simulink model "VFControl"  (R2017b)
settings: Solver=ode23tb  StartTime=0.0  StopTime=3  MaxStep=1e-4  RelTol=1e-3
undefined symbols (not defined in the file): DiscIntNeverNeededParam
libraries: simulink x5, powerlib x4
settings Model: Creator=80573  LastModifiedBy=80573
settings SolverCC: ZeroCrossAlgorithm=Adaptive
settings DebuggingCC: IgnoredZcDiagnostic=none

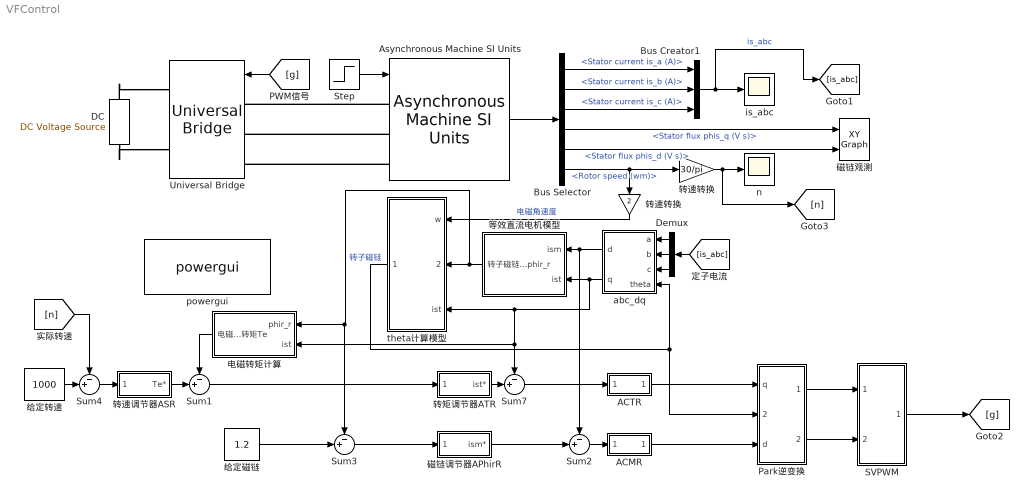
== system VFControl ==
  ACMR : Subsystem
  ACTR : Subsystem
  Asynchronous Machine SI Units : powerlib/Machines/Asynchronous Machine SI Units  RotorType=Squirrel-cage  PresetModel=No  MechanicalLoad=Torque Tm  ShowDetailedParameters=on  ReferenceFrame=Stationary  Units=SI  MeasurementBus=off  NominalParameters=[2200 380 50]  Stator=[0.435 0.002]  Rotor=[0.816 0.002]  Cage1=[0.4155 0.002066]  Cage2=[0.4168 0.0003495]  Lm=0.069  Mechanical=[0.19 0 2]  PolePairs=2  InitialConditions=[1 0 0 0 0 0 0 0]  SimulateSaturation=off  Saturation=[14.03593122, 27.81365428, 53.79336849, 72.68890987, 97.98006896, 148.6815601, 215.7428561, 302.9841135, 428.7778367 ; 230, 322, 414, 460, 506, 552, 598, 644, 690]  LoadFlowParameters=1492000  TsPowergui=0  TsBlock=-1  IterativeModel=Trapezoidal non iterative  IterativeDiscreteModel=Trapezoidal non iterative  Pmec=1.492e+006
  Bus Creator1 : BusCreator  Inputs=3
  Bus Selector : BusSelector  OutputSignals=Stator measurements.Stator current is_a (A),Stator measurements.Stator current is_b (A),Stator measurements.Stator current is_c (A),Stator measurements.Stator flux phis_q (V s),Stator measurements.Stator flux phis_d (V s),Mechanical.Rotor speed (wm)
  DC : powerlib/Electrical Sources/DC Voltage Source  Amplitude=510  Measurements=None
  Demux : Demux  Outputs=3
  Park逆变换 : Subsystem
  SVPWM : Subsystem
  Step : Step  Time=0.6  After=55  SampleTime=0
  Sum{1..4,7} (5 alike) : Sum  Inputs=-+|
  Universal Bridge : powerlib/Power Electronics/Universal Bridge  Arms=3  SnubberResistance=1e5  SnubberCapacitance=inf  Device=IGBT / Diodes  Ron=1e-3  Lon=0  ForwardVoltages="[  0  0  ]"  ForwardVoltage=0  GTOparameters=[ 10e-6 , 20e-6 ]  IGBTparameters=[ 1e-6 , 2e-6 ]  Measurements=None  Measurements_2=None  converterType=Rectifier
  abc_dq : Subsystem
  is_abc : Scope
  n : Scope
  powergui : powerlib/powergui  SimulationMode=Discrete  SampleTime=1e-5  frequency=50  Iterations=50  frequencyindice=50  Pbase=100e6  ErrMax=1e-4  UnitsV=kV  UnitsW=MW  buscounter=0  FunctionMessages=off  echomessages=off  EnableUseOfTLC=off  CurrentSourceSwitches=off  DisableSnubberDevices=off  DisableRonSwitches=off  DisableVfSwitches=off  DisplayEquations=off  SolverType=Tustin/Backward Euler (TBE)  Interpol=off  ExternalGateDelay=off  methode=off  Ts=100  x0status=zero  SPID=on  SwTol=0  HookPort=off  RestoreLinks=warning  ResistiveCurrentMeasurement=off  Frange=[0:2:500]  Ylog=off  Xlog=on  ShowGrid=off  save=off  variable=ZData  structure=0  ZoomFFT=on  StartTime=0.0  cycles=1  DisplayStyle=1  fundamental=60  FreqAxis=off  MaxFrequency=1000  frequencyindicesteady=1  RmsSteady=1  display=off
  theta计算模型 : Subsystem
  电磁转矩计算 : Subsystem
  磁链观测 : simulink/Sinks/XY Graph  xmin=-1  xmax=1  ymin=-1  ymax=1  st=-1
  磁链调节器APhirR : Subsystem
  等效直流电机模型 : Subsystem
  给定磁链 : Constant  Value=1.2
  给定转速 : Constant  Value=1000
  转矩调节器ATR : Subsystem
  转速调节器ASR : Subsystem
  转速转换 : Gain  Gain=30/pi
  "转速转换 " : Gain  Gain=2
  wires:
  Step/1 -> Asynchronous Machine SI Units/1
  "转速转换 "/1 -> theta计算模型/1(w)  "电磁角速度"
  转速转换/1 -> [n], n/1
  给定转速/1 -> Sum4/2
  [n] -> Sum4/1
  Sum1/1 -> 转矩调节器ATR/1(" ")
  theta计算模型/1(theta) -> Park逆变换/2(Theta), abc_dq/4(theta)
  Bus Selector/1 -> Bus Creator1/1  "<Stator current is_a (A)>"
  给定磁链/1 -> Sum3/2
  Bus Selector/4 -> 磁链观测/1  "<Stator flux phis_q (V s)>"
  转速调节器ASR/1(Te*) -> Sum1/2
  电磁转矩计算/1(电磁转矩Te) -> Sum1/1
  Demux/1 -> abc_dq/1(a)
  [is_abc] -> Demux/1
  等效直流电机模型/1(转子磁链phir_r) -> Sum3/1, 电磁转矩计算/1(phir_r), theta计算模型/2(phir_r)  "转子磁链"
  Bus Selector/5 -> 磁链观测/2  "<Stator flux phis_d (V s)>"
  Sum4/1 -> 转速调节器ASR/1("  ")
  [g] -> Universal Bridge/1
  Sum3/1 -> 磁链调节器APhirR/1(" ")
  Demux/2 -> abc_dq/2(b)
  Demux/3 -> abc_dq/3(c)
  SVPWM/1(PWM) -> [g]
  Bus Selector/3 -> Bus Creator1/3  "<Stator current is_c (A)>"
  abc_dq/2(q) -> Sum7/1, 电磁转矩计算/2(ist), theta计算模型/3(ist), 等效直流电机模型/2(ist)
  Bus Selector/6 -> 转速转换/1, "转速转换 "/1  "<Rotor speed (wm)>"
  Bus Selector/2 -> Bus Creator1/2  "<Stator current is_b (A)>"
  Asynchronous Machine SI Units/1 -> Bus Selector/1
  Bus Creator1/1 -> [is_abc], is_abc/1  "is_abc"
  abc_dq/1(d) -> Sum2/1, 等效直流电机模型/1(ism)
  转矩调节器ATR/1(ist*) -> Sum7/2
  磁链调节器APhirR/1(ism*) -> Sum2/2
  Sum2/1 -> ACMR/1("  ")
  Sum7/1 -> ACTR/1("  ")
  ACTR/1(" ") -> Park逆变换/1(q)
  ACMR/1(" ") -> Park逆变换/3(d)
  Park逆变换/1(alpha) -> SVPWM/1(Ualpha)
  Park逆变换/2(beta) -> SVPWM/2(Ubeta)
  connections:
  DC/LConn1 -- Universal Bridge/RConn2
  Asynchronous Machine SI Units/LConn3 -- Universal Bridge/LConn3
  DC/RConn1 -- Universal Bridge/RConn1
  Asynchronous Machine SI Units/LConn1 -- Universal Bridge/LConn1
  Asynchronous Machine SI Units/LConn2 -- Universal Bridge/LConn2

== system VFControl/ACMR ==
  "  " : Inport
  I积分放大倍数 : Gain  Gain=100
  PI输出限幅 : Saturate  UpperLimit=75  LowerLimit=-75
  P比例放大倍数 : Gain
  Scope : Scope  NumInputPorts=2
  Sum1 : Sum  Inputs=|++
  带限幅的连续积分 : Integrator  LimitOutput=on  UpperSaturationLimit=390  LowerSaturationLimit=-390
  " " : Outport
  wires:
  Sum1/1 -> PI输出限幅/1
  PI输出限幅/1 -> " "/1, Scope/1
  P比例放大倍数/1 -> Sum1/1
  I积分放大倍数/1 -> 带限幅的连续积分/1
  带限幅的连续积分/1 -> Scope/2, Sum1/2
  "  "/1 -> I积分放大倍数/1, P比例放大倍数/1

== system VFControl/ACTR ==
  "  " : Inport
  I积分放大倍数 : Gain  Gain=1200
  PI输出限幅 : Saturate  UpperLimit=380  LowerLimit=-380
  P比例放大倍数 : Gain  Gain=2
  Scope : Scope  NumInputPorts=2
  Sum1 : Sum  Inputs=|++
  带限幅的连续积分 : Integrator  LimitOutput=on  UpperSaturationLimit=400  LowerSaturationLimit=-400
  " " : Outport
  wires:
  Sum1/1 -> PI输出限幅/1
  PI输出限幅/1 -> " "/1, Scope/1
  P比例放大倍数/1 -> Sum1/1
  I积分放大倍数/1 -> 带限幅的连续积分/1
  带限幅的连续积分/1 -> Scope/2, Sum1/2
  "  "/1 -> I积分放大倍数/1, P比例放大倍数/1

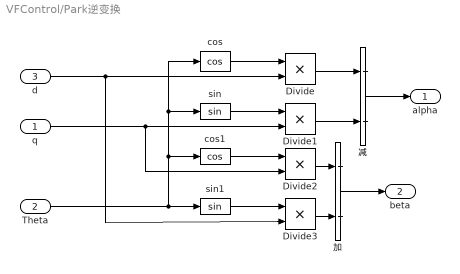
== system VFControl/Park逆变换 ==
  q : Inport
  Theta : Inport  Port=2
  d : Inport  Port=3
  Divide{,1..3} (4 alike) : Product  Inputs=**
  cos : Trigonometry  Operator=cos
  cos1 : Trigonometry  Operator=cos
  sin : Trigonometry
  sin1 : Trigonometry
  减 : Sum  Inputs=+-
  加 : Sum
  alpha : Outport
  beta : Outport  Port=2
  wires:
  sin/1 -> Divide1/1
  Divide2/1 -> 加/1
  cos1/1 -> Divide2/1
  cos/1 -> Divide/1
  Divide3/1 -> 加/2
  q/1 -> Divide2/2, Divide1/2
  Theta/1 -> cos/1, sin/1, cos1/1, sin1/1
  sin1/1 -> Divide3/1
  Divide1/1 -> 减/2
  Divide/1 -> 减/1
  d/1 -> Divide/2, Divide3/2
  加/1 -> beta/1
  减/1 -> alpha/1

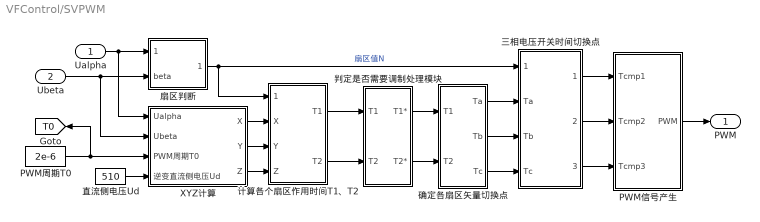
== system VFControl/SVPWM ==
  Ualpha : Inport
  Ubeta : Inport  Port=2
  PWM信号产生 : Subsystem
  PWM周期T0 : Constant  Value=2e-6
  XYZ计算 : Subsystem
  三相电压开关时间切换点 : Subsystem
  判定是否需要调制处理模块 : Subsystem
  扇区判断 : Subsystem
  直流侧电压Ud : Constant  Value=510
  确定各扇区矢量切换点 : Subsystem
  计算各个扇区作用时间T1、T2 : Subsystem
  PWM : Outport
  tag scope: T0=global
  wires:
  Ubeta/1 -> XYZ计算/2(Ubeta), 扇区判断/2(beta)
  Ualpha/1 -> XYZ计算/1(Ualpha), 扇区判断/1(alpha)
  PWM周期T0/1 -> XYZ计算/3(PWM周期T0), [T0]
  直流侧电压Ud/1 -> XYZ计算/4(逆变直流侧电压Ud)
  扇区判断/1(扇区值N) -> 计算各个扇区作用时间T1、T2/1(扇区值N), 三相电压开关时间切换点/1(扇区值N)  "扇区值N"
  XYZ计算/1(X) -> 计算各个扇区作用时间T1、T2/2(X)
  XYZ计算/2(Y) -> 计算各个扇区作用时间T1、T2/3(Y)
  XYZ计算/3(Z) -> 计算各个扇区作用时间T1、T2/4(Z)
  确定各扇区矢量切换点/2(Tb) -> 三相电压开关时间切换点/3(Tb)
  确定各扇区矢量切换点/3(Tc) -> 三相电压开关时间切换点/4(Tc)
  计算各个扇区作用时间T1、T2/2(T2) -> 判定是否需要调制处理模块/2(T2)
  计算各个扇区作用时间T1、T2/1(T1) -> 判定是否需要调制处理模块/1(T1)
  判定是否需要调制处理模块/2(T2*) -> 确定各扇区矢量切换点/2(T2)
  确定各扇区矢量切换点/1(Ta) -> 三相电压开关时间切换点/2(Ta)
  判定是否需要调制处理模块/1(T1*) -> 确定各扇区矢量切换点/1(T1)
  三相电压开关时间切换点/1(Tcmp1) -> PWM信号产生/1(Tcmp1)
  三相电压开关时间切换点/2(Tcmp2) -> PWM信号产生/2(Tcmp2)
  三相电压开关时间切换点/3(Tcmp3) -> PWM信号产生/3(Tcmp3)
  PWM信号产生/1(PWM) -> PWM/1

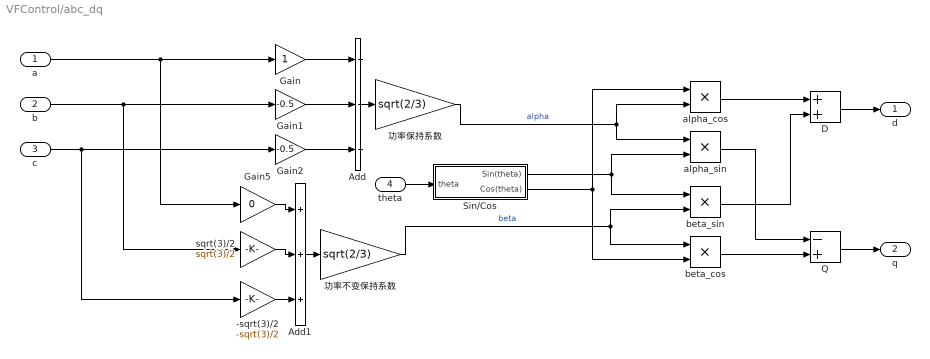
== system VFControl/abc_dq ==
  a : Inport
  b : Inport  Port=2
  c : Inport  Port=3
  theta : Inport  Port=4
  -sqrt(3)/2 : Gain  Gain=-sqrt(3)/2
  Add : Sum  Inputs=3
  Add1 : Sum  Inputs=3
  D : Sum
  Gain : Gain
  Gain1 : Gain  Gain=-0.5
  Gain2 : Gain  Gain=-0.5
  Gain5 : Gain  Gain=0
  Q : Sum  Inputs=-+
  Sin/Cos : Subsystem
  alpha_cos : Product
  alpha_sin : Product
  beta_cos : Product
  beta_sin : Product
  sqrt(3)/2 : Gain  Gain=sqrt(3)/2
  功率不变保持系数 : Gain  Gain=sqrt(2/3)
  功率保持系数 : Gain  Gain=sqrt(2/3)
  d : Outport
  q : Outport  Port=2
  wires:
  功率不变保持系数/1 -> beta_cos/1, beta_sin/2  "beta"
  D/1 -> d/1
  Sin/Cos/2(Cos(theta)) -> beta_cos/2, alpha_cos/1
  alpha_sin/1 -> Q/1
  Q/1 -> q/1
  beta_sin/1 -> D/2
  beta_cos/1 -> Q/2
  Sin/Cos/1(Sin(theta)) -> beta_sin/1, alpha_sin/2
  功率保持系数/1 -> alpha_cos/2, alpha_sin/1  "alpha"
  Add1/1 -> 功率不变保持系数/1
  c/1 -> Gain2/1, -sqrt(3)/2/1
  a/1 -> Gain5/1, Gain/1
  Gain2/1 -> Add/3
  sqrt(3)/2/1 -> Add1/2
  theta/1 -> Sin/Cos/1(theta)
  b/1 -> sqrt(3)/2/1, Gain1/1
  -sqrt(3)/2/1 -> Add1/3
  Gain1/1 -> Add/2
  Gain5/1 -> Add1/1
  alpha_cos/1 -> D/1
  Add/1 -> 功率保持系数/1
  Gain/1 -> Add/1

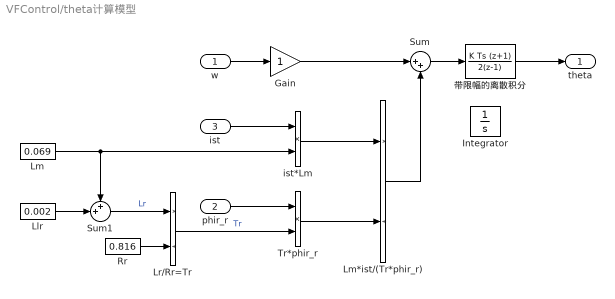
== system VFControl/theta计算模型 ==
  w : Inport
  phir_r : Inport  Port=2
  ist : Inport  Port=3
  Gain : Gain
  Integrator : Integrator
  Llr : Constant  Value=0.002
  Lm : Constant  Value=0.069
  Lm*ist/(Tr*phir_r) : Product  Inputs=*/
  Lr/Rr=Tr : Product  Inputs=*/
  Rr : Constant  Value=0.816
  Sum : Sum  Inputs=|++
  Sum1 : Sum  Inputs=++|
  Tr*phir_r : Product
  ist*Lm : Product
  带限幅的离散积分 : DiscreteIntegrator  IntegratorMethod=Integration: Trapezoidal  SampleTime=2e-5  LimitOutput=on  UpperSaturationLimit=3000  LowerSaturationLimit=-3000  ICPrevOutput=DiscIntNeverNeededParam  ICPrevScaledInput=DiscIntNeverNeededParam
  theta : Outport
  wires:
  ist*Lm/1 -> Lm*ist/(Tr*phir_r)/1
  Lm*ist/(Tr*phir_r)/1 -> Sum/2
  Sum/1 -> 带限幅的离散积分/1
  w/1 -> Gain/1
  带限幅的离散积分/1 -> theta/1
  Lr/Rr=Tr/1 -> Tr*phir_r/2  "Tr"
  Lm/1 -> Sum1/1, ist*Lm/2
  Tr*phir_r/1 -> Lm*ist/(Tr*phir_r)/2
  ist/1 -> ist*Lm/1
  phir_r/1 -> Tr*phir_r/1
  Rr/1 -> Lr/Rr=Tr/2
  Gain/1 -> Sum/1
  Sum1/1 -> Lr/Rr=Tr/1  "Lr"
  Llr/1 -> Sum1/2

== system VFControl/电磁转矩计算 ==
  phir_r : Inport
  ist : Inport  Port=2
  Llr : Constant  Value=0.002
  Lm : Constant  Value=0.069
  Sum1 : Sum  Inputs=++|
  ist*Lm*phir_r*np : Product  Inputs=4
  np : Constant  Value=2
  除法 : Product  Inputs=*/
  电磁转矩Te : Outport
  wires:
  np/1 -> ist*Lm*phir_r*np/4
  phir_r/1 -> ist*Lm*phir_r*np/3
  除法/1 -> 电磁转矩Te/1
  ist*Lm*phir_r*np/1 -> 除法/1
  Sum1/1 -> 除法/2  "Lr"
  Llr/1 -> Sum1/2
  ist/1 -> ist*Lm*phir_r*np/2
  Lm/1 -> Sum1/1, ist*Lm*phir_r*np/1

== system VFControl/磁链调节器APhirR ==
  " " : Inport
  I积分放大倍数 : Gain  Gain=100
  PI输出限幅 : Saturate  UpperLimit=13  LowerLimit=-13
  P比例放大倍数 : Gain  Gain=1.8
  Scope : Scope  NumInputPorts=2
  Sum1 : Sum  Inputs=|++
  带限幅的离散积分 : DiscreteIntegrator  SampleTime=2e-5  ICPrevOutput=DiscIntNeverNeededParam  ICPrevScaledInput=DiscIntNeverNeededParam
  带限幅的连续积分 : Integrator  LimitOutput=on  UpperSaturationLimit=15  LowerSaturationLimit=-15
  ism* : Outport
  wires:
  Sum1/1 -> PI输出限幅/1
  I积分放大倍数/1 -> 带限幅的连续积分/1
  P比例放大倍数/1 -> Sum1/1
  " "/1 -> I积分放大倍数/1, P比例放大倍数/1
  PI输出限幅/1 -> ism*/1, Scope/1
  带限幅的连续积分/1 -> Scope/2, Sum1/2

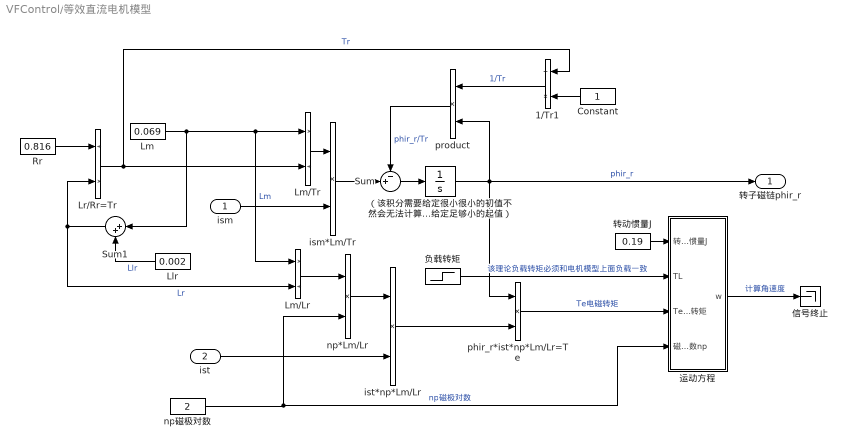
== system VFControl/等效直流电机模型 ==
  ism : Inport
  ist : Inport  Port=2
  1/Tr1 : Product  Inputs=/*
  Constant : Constant
  Llr : Constant  Value=0.002
  Lm : Constant  Value=0.069
  Lm/Lr : Product  Inputs=*/
  Lm/Tr : Product  Inputs=*/
  Lr/Rr=Tr : Product  Inputs=/*
  Rr : Constant  Value=0.816
  Sum : Sum  Inputs=-+|
  Sum1 : Sum  Inputs=|++
  ism*Lm/Tr : Product
  ist*np*Lm/Lr : Product
  np*Lm/Lr : Product
  np磁极对数 : Constant  Value=2
  phir_r*ist*np*Lm/Lr=Te : Product
  product : Product
  信号终止 : Terminator
  负载转矩 : Step  Time=0.6  After=55  SampleTime=0
  转动惯量J : Constant  Value=0.19
  运动方程 : Subsystem
  （该积分需要给定很小很小的初值不然会无法计算 原因是数学推导中积分起值为0所以一直都为0 所以要能够计算必须给定足够小的起值） : Integrator  InitialCondition=1e-5
  转子磁链phir_r : Outport
  wires:
  ism/1 -> ism*Lm/Tr/2
  Sum/1 -> （该积分需要给定很小很小的初值不然会无法计算 原因是数学推导中积分起值为0所以一直都为0 所以要能够计算必须给定足够小的起值）/1
  转动惯量J/1 -> 运动方程/1(转动惯量J)
  运动方程/1(w) -> 信号终止/1  "计算角速度"
  phir_r*ist*np*Lm/Lr=Te/1 -> 运动方程/3(Te电磁转矩)  "Te电磁转矩"
  负载转矩/1 -> 运动方程/2(TL)  "该理论负载转矩必须和电机模型上面负载一致"
  np*Lm/Lr/1 -> ist*np*Lm/Lr/1
  Lm/1 -> Sum1/1, Lm/Lr/1, Lm/Tr/1  "Lm"
  Lm/Tr/1 -> ism*Lm/Tr/1
  ist*np*Lm/Lr/1 -> phir_r*ist*np*Lm/Lr=Te/2
  ism*Lm/Tr/1 -> Sum/2
  product/1 -> Sum/1  "phir_r/Tr"
  ist/1 -> ist*np*Lm/Lr/2
  np磁极对数/1 -> np*Lm/Lr/2, 运动方程/4(磁极对数np)  "np磁极对数"
  Lm/Lr/1 -> np*Lm/Lr/1
  （该积分需要给定很小很小的初值不然会无法计算 原因是数学推导中积分起值为0所以一直都为0 所以要能够计算必须给定足够小的起值）/1 -> 转子磁链phir_r/1, product/2, phir_r*ist*np*Lm/Lr=Te/1  "phir_r"
  1/Tr1/1 -> product/1  "1/Tr"
  Lr/Rr=Tr/1 -> Lm/Tr/2, 1/Tr1/1  "Tr"
  Rr/1 -> Lr/Rr=Tr/1
  Constant/1 -> 1/Tr1/2
  Sum1/1 -> Lm/Lr/2, Lr/Rr=Tr/2  "Lr"
  Llr/1 -> Sum1/2  "Llr"

== system VFControl/转矩调节器ATR ==
  " " : Inport
  I积分放大倍数 : Gain  Gain=12
  PI输出限幅 : Saturate  UpperLimit=60  LowerLimit=-60
  P比例放大倍数 : Gain  Gain=4.5
  Scope : Scope  NumInputPorts=2
  Sum3 : Sum  Inputs=|++
  带限幅的离散积分 : DiscreteIntegrator  SampleTime=2e-5  ICPrevOutput=DiscIntNeverNeededParam  ICPrevScaledInput=DiscIntNeverNeededParam
  带限幅的连续积分 : Integrator  LimitOutput=on  UpperSaturationLimit=65  LowerSaturationLimit=-65
  ist* : Outport
  wires:
  Sum3/1 -> PI输出限幅/1
  P比例放大倍数/1 -> Sum3/1
  " "/1 -> I积分放大倍数/1, P比例放大倍数/1
  I积分放大倍数/1 -> 带限幅的连续积分/1
  PI输出限幅/1 -> ist*/1, Scope/1
  带限幅的连续积分/1 -> Scope/2, Sum3/2

== system VFControl/转速调节器ASR ==
  "  " : Inport
  I积分放大倍数 : Gain  Gain=0.8
  PI输出限幅 : Saturate  UpperLimit=75  LowerLimit=-75
  P比例放大倍数 : Gain  Gain=5
  Scope : Scope  NumInputPorts=2
  Sum1 : Sum  Inputs=|++
  带限幅的连续积分 : Integrator  LimitOutput=on  UpperSaturationLimit=80  LowerSaturationLimit=-80
  Te* : Outport
  wires:
  Sum1/1 -> PI输出限幅/1
  PI输出限幅/1 -> Te*/1, Scope/1
  P比例放大倍数/1 -> Sum1/1
  I积分放大倍数/1 -> 带限幅的连续积分/1
  带限幅的连续积分/1 -> Scope/2, Sum1/2
  "  "/1 -> I积分放大倍数/1, P比例放大倍数/1

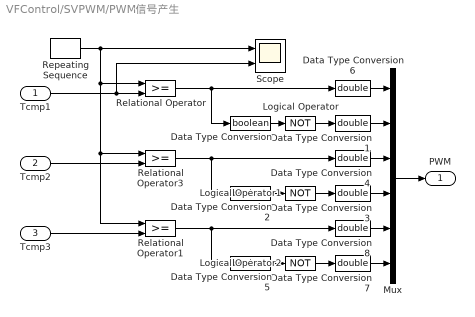
== system VFControl/SVPWM/PWM信号产生 ==
  Tcmp1 : Inport
  Tcmp2 : Inport  Port=2
  Tcmp3 : Inport  Port=3
  Data Type Conversion : DataTypeConversion  OutDataTypeStr=boolean
  Data Type Conversion{1,3..4,6..8} (6 alike) : DataTypeConversion  OutDataTypeStr=double
  Data Type Conversion2 : DataTypeConversion  OutDataTypeStr=boolean
  Data Type Conversion5 : DataTypeConversion  OutDataTypeStr=boolean
  Logical Operator : Logic  Operator=NOT  AllPortsSameDT=off  OutDataTypeStr=boolean
  Logical Operator1 : Logic  Operator=NOT  AllPortsSameDT=off  OutDataTypeStr=boolean
  Logical Operator2 : Logic  Operator=NOT  AllPortsSameDT=off  OutDataTypeStr=boolean
  Mux : Mux  Inputs=6
  Relational Operator : RelationalOperator  OutDataTypeStr=boolean  RndMeth=Nearest
  Relational Operator1 : RelationalOperator  OutDataTypeStr=boolean  RndMeth=Nearest
  Relational Operator3 : RelationalOperator  OutDataTypeStr=boolean  RndMeth=Nearest
  Repeating Sequence : simulink/Sources/Repeating Sequence  rep_seq_t=[0 1e-4 2e-4]  rep_seq_y=[0 1.3e-6 0]
  Scope : Scope  NumInputPorts=2
  PWM : Outport
  wires:
  Data Type Conversion/1 -> Logical Operator/1
  Logical Operator/1 -> Data Type Conversion1/1
  Relational Operator/1 -> Data Type Conversion6/1, Data Type Conversion/1
  Logical Operator1/1 -> Data Type Conversion3/1
  Relational Operator3/1 -> Data Type Conversion4/1, Data Type Conversion2/1
  Data Type Conversion2/1 -> Logical Operator1/1
  Relational Operator1/1 -> Data Type Conversion8/1, Data Type Conversion5/1
  Data Type Conversion5/1 -> Logical Operator2/1
  Logical Operator2/1 -> Data Type Conversion7/1
  Repeating Sequence/1 -> Relational Operator1/1, Relational Operator3/1, Relational Operator/1, Scope/1
  Tcmp1/1 -> Scope/2, Relational Operator/2
  Tcmp2/1 -> Relational Operator3/2
  Tcmp3/1 -> Relational Operator1/2
  Data Type Conversion6/1 -> Mux/1
  Data Type Conversion1/1 -> Mux/2
  Data Type Conversion4/1 -> Mux/3
  Data Type Conversion3/1 -> Mux/4
  Data Type Conversion8/1 -> Mux/5
  Data Type Conversion7/1 -> Mux/6
  Mux/1 -> PWM/1

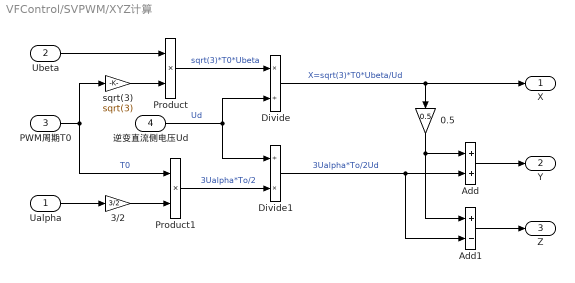
== system VFControl/SVPWM/XYZ计算 ==
  Ualpha : Inport
  Ubeta : Inport  Port=2
  PWM周期T0 : Inport  Port=3
  逆变直流侧电压Ud : Inport  Port=4
  0.5 : Gain  Gain=0.5
  3/2 : Gain  Gain=3/2
  Add : Sum
  Add1 : Sum  Inputs=+-
  Divide : Product  Inputs=*/
  Divide1 : Product  Inputs=/*
  Product : Product
  Product1 : Product
  "sqrt(3) " : Gain  Gain=sqrt(3)
  X : Outport
  Y : Outport  Port=2
  Z : Outport  Port=3
  wires:
  Divide/1 -> 0.5/1, X/1  "X=sqrt(3)*T0*Ubeta/Ud"
  Product/1 -> Divide/1  "sqrt(3)*T0*Ubeta"
  逆变直流侧电压Ud/1 -> Divide1/1, Divide/2  "Ud"
  Ualpha/1 -> 3/2/1
  Divide1/1 -> Add1/2, Add/2  "3Ualpha*To/2Ud"
  Add/1 -> Y/1
  Ubeta/1 -> Product/1
  3/2/1 -> Product1/2
  Product1/1 -> Divide1/2  "3Ualpha*To/2"
  "sqrt(3) "/1 -> Product/2
  PWM周期T0/1 -> "sqrt(3) "/1, Product1/1  "T0"
  Add1/1 -> Z/1
  0.5/1 -> Add/1, Add1/1

== system VFControl/SVPWM/三相电压开关时间切换点 ==
  扇区值N : Inport
  Ta : Inport  Port=2
  Tb : Inport  Port=3
  Tc : Inport  Port=4
  Multiport Switch : MultiPortSwitch  Inputs=6  OutDataTypeStr=double
  Multiport Switch1 : MultiPortSwitch  Inputs=6  OutDataTypeStr=double
  Multiport Switch2 : MultiPortSwitch  Inputs=6  OutDataTypeStr=double
  Tcmp1 : Outport
  Tcmp2 : Outport  Port=2
  Tcmp3 : Outport  Port=3
  wires:
  扇区值N/1 -> Multiport Switch2/1, Multiport Switch1/1, Multiport Switch/1  "扇区选择"
  Multiport Switch/1 -> Tcmp1/1
  Multiport Switch1/1 -> Tcmp2/1
  Multiport Switch2/1 -> Tcmp3/1
  Ta/1 -> Multiport Switch/4, Multiport Switch2/7, Multiport Switch2/5, Multiport Switch1/6, Multiport Switch1/2, Multiport Switch/3
  Tb/1 -> Multiport Switch2/6, Multiport Switch2/3, Multiport Switch1/5, Multiport Switch1/4, Multiport Switch/7, Multiport Switch/2
  Tc/1 -> Multiport Switch1/7, Multiport Switch2/2, Multiport Switch2/4, Multiport Switch1/3, Multiport Switch/6, Multiport Switch/5

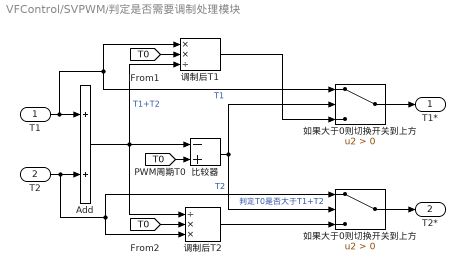
== system VFControl/SVPWM/判定是否需要调制处理模块 ==
  T1 : Inport
  T2 : Inport  Port=2
  Add : Sum
  如果大于0则切换开关到上方 : Switch  Criteria=u2 > Threshold
  "如果大于0则切换开关到上方 " : Switch  Criteria=u2 > Threshold
  比较器 : Sum  Inputs=-+
  调制后T1 : Product  Inputs=**/
  调制后T2 : Product  Inputs=/**
  T1* : Outport
  T2* : Outport  Port=2
  wires:
  如果大于0则切换开关到上方/1 -> T1*/1
  "如果大于0则切换开关到上方 "/1 -> T2*/1
  T2/1 -> "如果大于0则切换开关到上方 "/1, 调制后T2/3, Add/2  "T2"
  T1/1 -> 如果大于0则切换开关到上方/1, 调制后T1/1, Add/1  "T1"
  [T0] -> 比较器/2
  Add/1 -> 调制后T2/1, 比较器/1, 调制后T1/3  "T1+T2"
  比较器/1 -> "如果大于0则切换开关到上方 "/2, 如果大于0则切换开关到上方/2  "判定T0是否大于T1+T2"
  调制后T2/1 -> "如果大于0则切换开关到上方 "/3
  调制后T1/1 -> 如果大于0则切换开关到上方/3
  [T0] -> 调制后T1/2
  [T0] -> 调制后T2/2

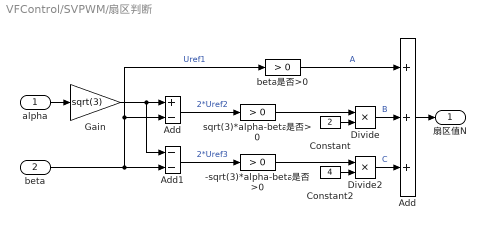
== system VFControl/SVPWM/扇区判断 ==
  alpha : Inport
  beta : Inport  Port=2
  -sqrt(3)*alpha-beta是否>0 : simulink/Logic and Bit Operations/Compare To Zero  relop=>  OutDataTypeStr=boolean
  Add : Sum  Inputs=+-
  "Add " : Sum  Inputs=+++
  Add1 : Sum  Inputs=--
  Constant : Constant  Value=2
  Constant2 : Constant  Value=4
  Divide : Product  Inputs=**
  Divide2 : Product  Inputs=**
  Gain : Gain  Gain=sqrt(3)
  beta是否>0 : simulink/Logic and Bit Operations/Compare To Zero  relop=>  OutDataTypeStr=boolean
  sqrt(3)*alpha-beta是否>0 : simulink/Logic and Bit Operations/Compare To Zero  relop=>  OutDataTypeStr=boolean
  扇区值N : Outport
  wires:
  beta/1 -> Add1/2, Add/2, beta是否>0/1  "Uref1"
  alpha/1 -> Gain/1
  Gain/1 -> Add/1, Add1/1
  Add/1 -> sqrt(3)*alpha-beta是否>0/1  "2*Uref2"
  Add1/1 -> -sqrt(3)*alpha-beta是否>0/1  "2*Uref3"
  -sqrt(3)*alpha-beta是否>0/1 -> Divide2/1
  sqrt(3)*alpha-beta是否>0/1 -> Divide/1
  Constant/1 -> Divide/2
  Constant2/1 -> Divide2/2
  beta是否>0/1 -> "Add "/1  "A"
  Divide/1 -> "Add "/2  "B"
  Divide2/1 -> "Add "/3  "C"
  "Add "/1 -> 扇区值N/1

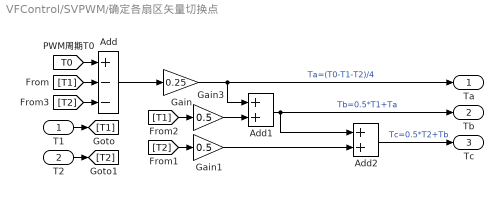
== system VFControl/SVPWM/确定各扇区矢量切换点 ==
  T1 : Inport
  T2 : Inport  Port=2
  Add : Sum  Inputs=+--
  Add1 : Sum
  Add2 : Sum
  Gain : Gain  Gain=0.25
  Gain1 : Gain  Gain=0.5
  Gain3 : Gain  Gain=0.5
  Ta : Outport
  Tb : Outport  Port=2
  Tc : Outport  Port=3
  wires:
  Gain/1 -> Ta/1, Add1/1  "Ta=(T0-T1-T2)/4"
  [T0] -> Add/1
  Add/1 -> Gain/1
  Add1/1 -> Tb/1, Add2/1  "Tb=0.5*T1+Ta"
  Add2/1 -> Tc/1  "Tc=0.5*T2+Tb"
  Gain3/1 -> Add1/2
  Gain1/1 -> Add2/2
  T1/1 -> [T1]
  [T1] -> Add/2
  T2/1 -> [T2]
  [T1] -> Gain3/1
  [T2] -> Gain1/1
  [T2] -> Add/3

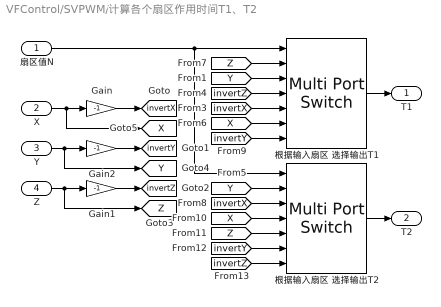
== system VFControl/SVPWM/计算各个扇区作用时间T1、T2 ==
  扇区值N : Inport
  X : Inport  Port=2
  Y : Inport  Port=3
  Z : Inport  Port=4
  Gain : Gain  Gain=-1
  Gain1 : Gain  Gain=-1
  Gain2 : Gain  Gain=-1
  根据输入扇区 选择输出T1 : MultiPortSwitch  Inputs=6
  根据输入扇区 选择输出T2 : MultiPortSwitch  Inputs=6
  T1 : Outport
  T2 : Outport  Port=2
  tag scope: X=global, Y=global, Z=global, invertX=global, invertY=global, invertZ=global
  wires:
  Z/1 -> [Z], Gain1/1
  X/1 -> [X], Gain/1
  扇区值N/1 -> 根据输入扇区 选择输出T2/1, 根据输入扇区 选择输出T1/1
  根据输入扇区 选择输出T2/1 -> T2/1
  根据输入扇区 选择输出T1/1 -> T1/1
  Y/1 -> [Y], Gain2/1
  Gain/1 -> [invertX]
  Gain2/1 -> [invertY]
  Gain1/1 -> [invertZ]
  [Z] -> 根据输入扇区 选择输出T1/2
  [Y] -> 根据输入扇区 选择输出T2/2
  [Y] -> 根据输入扇区 选择输出T1/3
  [invertX] -> 根据输入扇区 选择输出T2/3
  [invertZ] -> 根据输入扇区 选择输出T1/4
  [invertX] -> 根据输入扇区 选择输出T1/5
  [X] -> 根据输入扇区 选择输出T1/6
  [invertY] -> 根据输入扇区 选择输出T1/7
  [X] -> 根据输入扇区 选择输出T2/4
  [Z] -> 根据输入扇区 选择输出T2/5
  [invertY] -> 根据输入扇区 选择输出T2/6
  [invertZ] -> 根据输入扇区 选择输出T2/7

== system VFControl/abc_dq/Sin//Cos ==
  theta : Inport
  cos : Trigonometry  Operator=cos
  sin : Trigonometry
  Sin(theta) : Outport
  Cos(theta) : Outport  Port=2
  wires:
  sin/1 -> Sin(theta)/1
  theta/1 -> sin/1, cos/1
  cos/1 -> Cos(theta)/1

== system VFControl/等效直流电机模型/运动方程 ==
  转动惯量J : Inport
  TL : Inport  Port=2
  Te电磁转矩 : Inport  Port=3
  磁极对数np : Inport  Port=4
  Sum1 : Sum  Inputs=|+-
  dw/dt : Product
  np/J : Product  Inputs=*/
  积分 : Integrator
  w : Outport
  wires:
  转动惯量J/1 -> np/J/2
  Sum1/1 -> dw/dt/2
  TL/1 -> Sum1/2
  积分/1 -> w/1
  磁极对数np/1 -> np/J/1
  np/J/1 -> dw/dt/1
  Te电磁转矩/1 -> Sum1/1
  dw/dt/1 -> 积分/1
